simulink model "es3_sim"  (Simulink 7.9)
settings: Solver=ode45  StartTime=0.0  StopTime=10  RelTol=1e-3
values from neighbouring files (symbols this model uses):
  A = [3 1;5 2]    [es3.m]
  B = [1;0]    [es3.m]
  C = [1 0]    [es3.m]
  K = place(A,B,autoval)    [es3.m]
  ueq = 1    [es3.m]
  x0 = [1 1]    [es3.m]
  xeq = -inv(A)*B*ueq    [es3.m]
settings Model: Creator=claudio  LastModifiedBy=patrizio
settings OptimizationCC: InlineInvariantSignals=on  InitFltsAndDblsToZero=on
settings DebuggingCC: SaveWithParameterizedLinksMsg=none  SignalResolutionControl=TryResolveAllWithWarning  MultiTaskDSMMsg=warning  MultiTaskCondExecSysMsg=none  FcnCallInpInsideContextMsg=Use local settings  StrictBusMsg=None
settings RTWCC: IncludeERTFirstTime=on
settings GRTTargetCC: TargetFcnLib=ansi_tfl_tmw.mat  CombineOutputUpdateFcns=off  GRTInterface=on

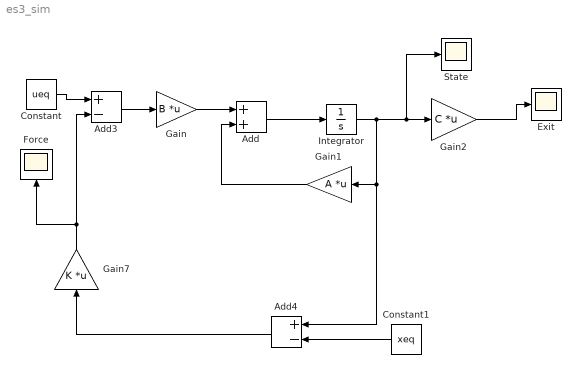
== system es3_sim ==
  Add : Sum
  Add3 : Sum  Inputs=+-
  Add4 : Sum  Inputs=+-
  Constant : Constant  Value=ueq
  Constant1 : Constant  Value=xeq
  Exit : Scope
  Force : Scope
      settings: SaveName=ScopeData4
  Gain : Gain  Gain=B  Multiplication=Matrix(K*u)
  Gain1 : Gain  Gain=A  Multiplication=Matrix(K*u)
  Gain2 : Gain  Gain=C  Multiplication=Matrix(K*u)
  Gain7 : Gain  Gain=K  Multiplication=Matrix(K*u)
  Integrator : Integrator  InitialCondition=x0
  State : Scope
      settings: SaveName=ScopeData3
  wires:
  Add/1 -> Integrator/1
  Gain/1 -> Add/1
  Integrator/1 -> Gain2/1, State/1, Gain1/1, Add4/1
  Gain1/1 -> Add/2
  Gain2/1 -> Exit/1
  Add3/1 -> Gain/1
  Constant/1 -> Add3/1
  Gain7/1 -> Add3/2, Force/1
  Constant1/1 -> Add4/2
  Add4/1 -> Gain7/1
